simulink model "MagnetSystem"  (R2020b)
settings: Solver=VariableStepAuto  StartTime=0.0  StopTime=10  FixedStep=0.001  RelTol=1e-3
values from neighbouring files (symbols this model uses):
  A = [0, dfdx/m, dfdi/m ... (first row only)    [magnetABCD.m]
  B = [0 ... (first row only)    [magnetABCD.m]
  C = zeros(2,3)    [magnetABCD.m]
  x0 = positionConversion(equilibrium{ncards, 4})    [equilibriumFeatures.m]
undefined symbols (not defined in the file or in its folder): coeffLQR, coeffPP, current, F, initialConditions, initialConditionsOBS, intensityVariance, kdp, kic, kip, KoK, KoLQR, kpc, kpp, LL, positions, positionsVariance, target
libraries: simulink x1
settings Model: Creator=paolo  LastModifiedBy=paolo

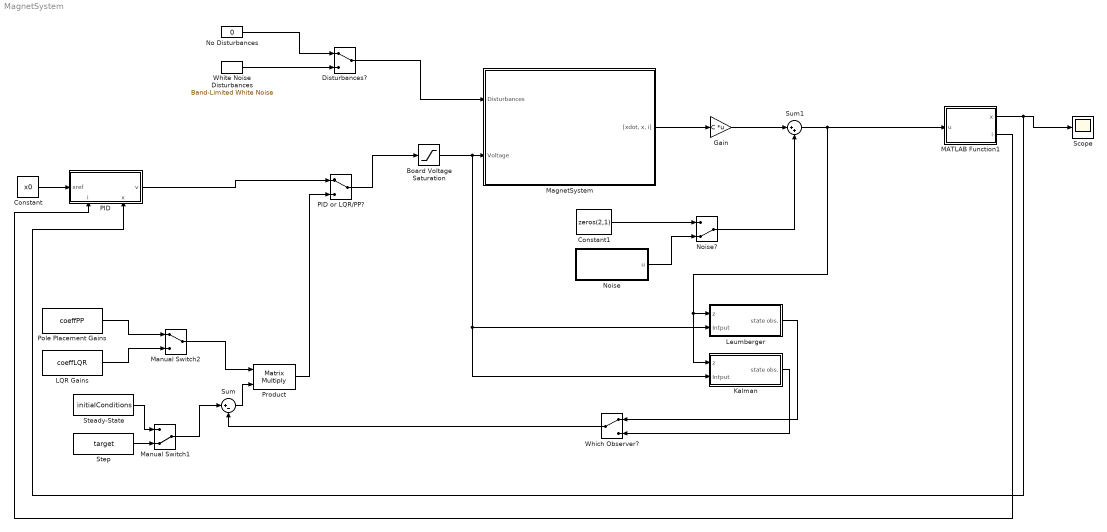
== system MagnetSystem ==
  Board Voltage Saturation : Saturate  UpperLimit=15  LowerLimit=0.1
  Constant : Constant  Value=x0
  Constant1 : Constant  Value=zeros(2,1)
  Disturbances? : ManualSwitch
  Gain : Gain  Gain=C  Multiplication=Matrix(K*u)
  Kalman : Subsystem
  LQR Gains : Constant  Value=coeffLQR  VectorParams1D=off
  Leumberger : Subsystem
  MATLAB Function1 : MATLAB Function  TreatAsAtomicUnit=on
  MagnetSystem : Subsystem
  Manual Switch1 : ManualSwitch  CurrentSetting=0
  Manual Switch2 : ManualSwitch
  No Disturbances : Constant  Value=0
  Noise : Subsystem
  Noise? : ManualSwitch  CurrentSetting=0
  PID : Subsystem
      settings: PortSchema="{\"entries\":[{\"content\":{\"sides\":[{\"content\":{\"connectorIds\":[\"In1\"]},\"type\":\"ConnectorPlacement.EquallySpacedRectSide\",\"uuid\":\"14521f87-e048-4244-bdcc-908d8d88763b\"},{\"content\":{\"connectorIds\":[\"Out1\"],\"side\":\"RIGHT\"},\"type\":\"ConnectorPlacement.EquallySpacedRectSide\",\"uuid\":\"c5527259-ae1a-43ba-91f2-6df4aeebe36b\"},{\"content\":{\"connectorIds\":[],\"side\":\"TOP\"},\"type\":\"ConnectorPlacement.EquallySpacedRectSide\",\"uuid\":\"73278f71-19a1-45c2-a1b8-f0fc113770d2\"},{\"content\":{\"connectorIds\":[\"In2\",\"In3\"],\"side\":\"BOTTOM\"},\"type\":\"ConnectorPlacement.EquallySpacedRectSide\",\"uuid\":\"a0ac4a62-b9ad-495a-a277-bc45d4b1109c\"},{\"content\":{\"connectorIds\":[],\"side\":\"HIDDEN\"},\"type\":\"ConnectorPlacement.EquallySpacedRectSide\",\"uuid\":\"850a1bc1-7bbe-470b-baa6-7596bfe1b42b\"}]},\"type\":\"ConnectorPlacement.EquallySpacedConnector\",\"uuid\":\"f2c623c1-bb11-4af5-93db-0114832c2495\"}],\"packageUris\":[\"http://schema.mathworks.com/mf0/Connector/R2020b\"],\"version\":\"1.0\"}"
  PID or LQR/PP? : ManualSwitch
  Pole Placement Gains : Constant  Value=coeffPP  VectorParams1D=off
  Product : Product  Multiplication=Matrix(*)
  Scope : Scope
  Steady-State : Constant  Value=initialConditions  VectorParams1D=off
  Step : Constant  Value=target  VectorParams1D=off
  Sum : Sum  Inputs=|+-
  Sum1 : Sum  Inputs=|++
  Which Observer? : ManualSwitch
  White Noise Disturbances : simulink/Sources/Band-Limited White Noise  Cov=[0.1]  Ts=0.1  seed=[23341]
  wires:
  Board Voltage Saturation/1 -> Kalman/2(Intput), Leumberger/2(Intput), MagnetSystem/2(Voltage)
  MagnetSystem/1("[xdot, x, i]") -> Gain/1
  Steady-State/1 -> Manual Switch1/1
  Sum/1 -> Product/2
  No Disturbances/1 -> Disturbances?/1
  Disturbances?/1 -> MagnetSystem/1(Disturbances)
  White Noise Disturbances/1 -> Disturbances?/2
  Step/1 -> Manual Switch1/2
  Manual Switch1/1 -> Sum/1
  Product/1 -> PID or LQR/PP?/2
  PID or LQR/PP?/1 -> Board Voltage Saturation/1
  PID/1(v) -> PID or LQR/PP?/1
  Constant/1 -> PID/1(xref)
  Manual Switch2/1 -> Product/1
  LQR Gains/1 -> Manual Switch2/2
  Pole Placement Gains/1 -> Manual Switch2/1
  Leumberger/1(state obs.) -> Which Observer?/1
  Kalman/1(state obs.) -> Which Observer?/2
  Which Observer?/1 -> Sum/2
  Gain/1 -> Sum1/1
  MATLAB Function1/1(x) -> PID/3(x), Scope/1
  Noise?/1 -> Sum1/2
  Noise/1(u) -> Noise?/2
  Sum1/1 -> Kalman/1(z), Leumberger/1(z), MATLAB Function1/1(u)
  Constant1/1 -> Noise?/1
  MATLAB Function1/2(i) -> PID/2(i)

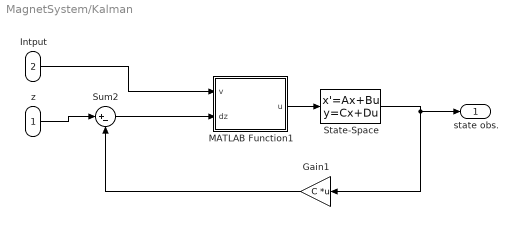
== system MagnetSystem/Kalman ==
  z : Inport
  Intput : Inport  Port=2
  Gain1 : Gain  Gain=C  Multiplication=Matrix(K*u)
  MATLAB Function1 : MATLAB Function  TreatAsAtomicUnit=on
  State-Space : StateSpace  A=A  B=[B KoK]  C=eye(3)  D=zeros(3,3)  InitialCondition=initialConditionsOBS
  Sum2 : Sum  Inputs=|+-
  state obs. : Outport
  wires:
  z/1 -> Sum2/1
  State-Space/1 -> Gain1/1, state obs./1
  Gain1/1 -> Sum2/2
  Sum2/1 -> MATLAB Function1/2(dz)
  Intput/1 -> MATLAB Function1/1(v)
  MATLAB Function1/1(u) -> State-Space/1

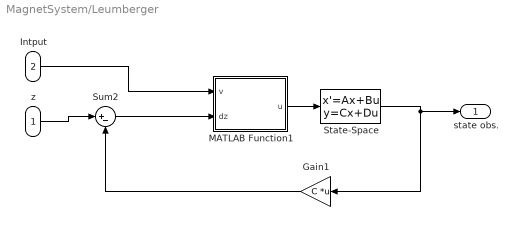
== system MagnetSystem/Leumberger ==
  z : Inport
  Intput : Inport  Port=2
  Gain1 : Gain  Gain=C  Multiplication=Matrix(K*u)
  MATLAB Function1 : MATLAB Function  TreatAsAtomicUnit=on
  State-Space : StateSpace  A=A  B=[B KoLQR]  C=eye(3)  D=zeros(3,3)  InitialCondition=initialConditionsOBS
  Sum2 : Sum  Inputs=|+-
  state obs. : Outport
  wires:
  z/1 -> Sum2/1
  State-Space/1 -> Gain1/1, state obs./1
  Gain1/1 -> Sum2/2
  Sum2/1 -> MATLAB Function1/2(dz)
  Intput/1 -> MATLAB Function1/1(v)
  MATLAB Function1/1(u) -> State-Space/1

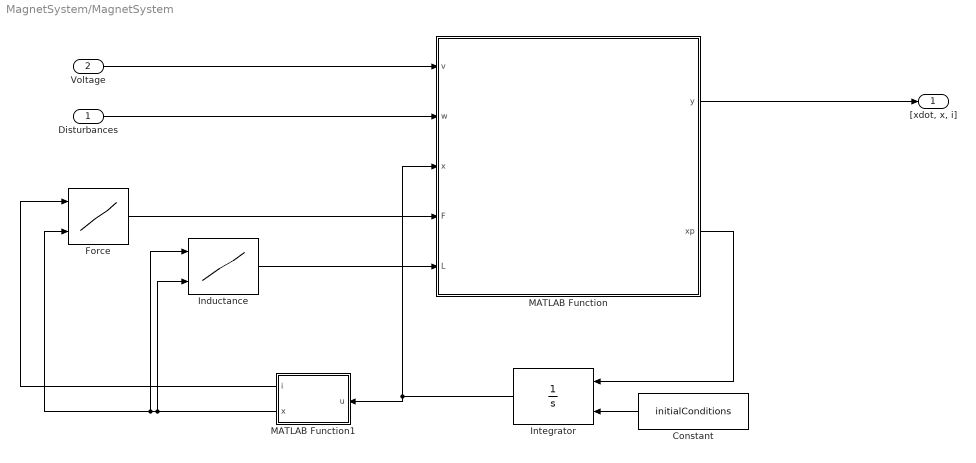
== system MagnetSystem/MagnetSystem ==
  Disturbances : Inport
  Voltage : Inport  Port=2
  Constant : Constant  Value=initialConditions
  Force : Lookup_n-D  BreakpointsForDimension1=current  BreakpointsForDimension2=positions  Table=F  InternalRulePriority=Speed  RndMeth=Simplest  InputSameDT=on
      settings: InputPortMap=u0,u1
  Inductance : Lookup_n-D  BreakpointsForDimension1=current  BreakpointsForDimension2=positions  Table=LL  InternalRulePriority=Speed  RndMeth=Simplest  InputSameDT=on
      settings: InputPortMap=u0,u1
  Integrator : Integrator  InitialConditionSource=external
  MATLAB Function : MATLAB Function  TreatAsAtomicUnit=on
  MATLAB Function1 : MATLAB Function  TreatAsAtomicUnit=on
  "[xdot, x, i]" : Outport
  wires:
  Integrator/1 -> MATLAB Function1/1(u), MATLAB Function/3(x)
  Voltage/1 -> MATLAB Function/1(v)
  Constant/1 -> Integrator/2
  Disturbances/1 -> MATLAB Function/2(w)
  MATLAB Function/1(y) -> "[xdot, x, i]"/1
  MATLAB Function/2(xp) -> Integrator/1
  MATLAB Function1/1(i) -> Force/1
  MATLAB Function1/2(x) -> Inductance/2, Force/2, Inductance/1
  Inductance/1 -> MATLAB Function/5(L)
  Force/1 -> MATLAB Function/4(F)

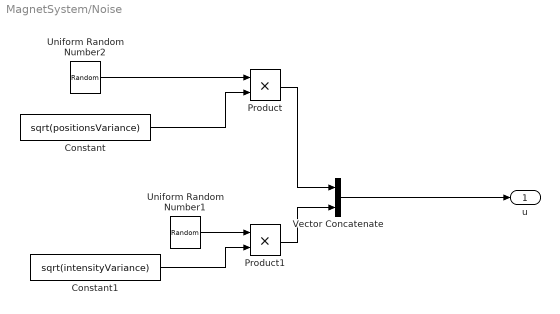
== system MagnetSystem/Noise ==
  Constant : Constant  Value=sqrt(positionsVariance)
  Constant1 : Constant  Value=sqrt(intensityVariance)
  Product : Product
  Product1 : Product
  Uniform Random Number1 : UniformRandomNumber  SampleTime=0.001
  Uniform Random Number2 : UniformRandomNumber  SampleTime=0.001
  Vector Concatenate : Concatenate  Mode=Multidimensional array
  u : Outport
  wires:
  Constant1/1 -> Product1/2
  Vector Concatenate/1 -> u/1
  Constant/1 -> Product/2
  Product1/1 -> Vector Concatenate/2
  Product/1 -> Vector Concatenate/1
  Uniform Random Number2/1 -> Product/1
  Uniform Random Number1/1 -> Product1/1

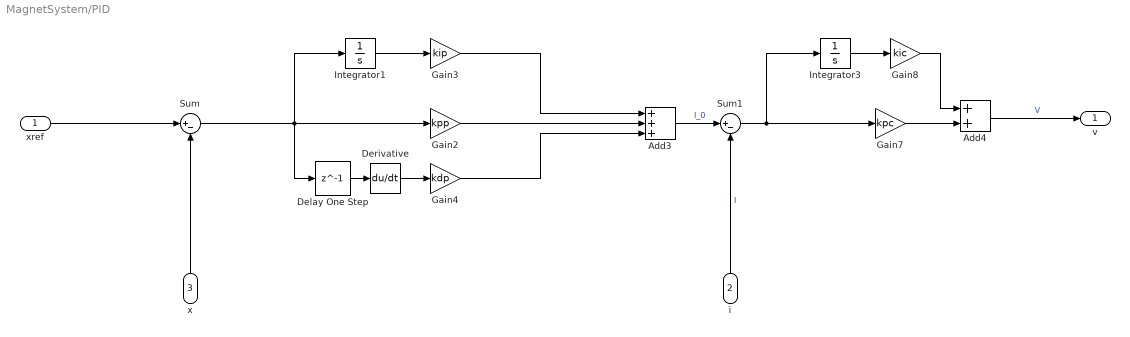
== system MagnetSystem/PID ==
  xref : Inport
  i : Inport  Port=2
  x : Inport  Port=3
  Add3 : Sum  Inputs=+++
  Add4 : Sum
  Delay One Step : Delay  DelayLength=1
  Derivative : Derivative
  Gain2 : Gain  Gain=kpp
  Gain3 : Gain  Gain=kip
  Gain4 : Gain  Gain=kdp
  Gain7 : Gain  Gain=kpc
  Gain8 : Gain  Gain=kic
  Integrator1 : Integrator
  Integrator3 : Integrator
  Sum : Sum  Inputs=|+-
  Sum1 : Sum  Inputs=|+-
  v : Outport
  wires:
  Sum/1 -> Integrator1/1, Delay One Step/1, Gain2/1
  Add4/1 -> v/1  "V"
  Gain4/1 -> Add3/3
  Derivative/1 -> Gain4/1
  i/1 -> Sum1/2  "I"
  Gain3/1 -> Add3/1
  Add3/1 -> Sum1/1  "I_0"
  Gain2/1 -> Add3/2
  Gain7/1 -> Add4/2
  Sum1/1 -> Integrator3/1, Gain7/1
  Gain8/1 -> Add4/1
  Integrator1/1 -> Gain3/1
  Integrator3/1 -> Gain8/1
  xref/1 -> Sum/1
  x/1 -> Sum/2
  Delay One Step/1 -> Derivative/1

== matlab function MagnetSystem/MATLAB Function1 ==
  data: i output; u input; x output
function [i, x] = fcn(u)
x = u(2);
i = u(3);

== matlab function MagnetSystem/MATLAB Function ==
  data: v input; y output; w input; x input; xp output; F input; L input
function [y,xp] = fcn(v,w,x,F,L)

R = 4.1;
m = 0.8766;
g = 9.81;

x1 = x(1);
x2 = x(2);
x3 = x(3);

xp = [((F/m)-g);x1;((v+w)-R*x3)/L];
y = [x1;x2;x3];

== matlab function MagnetSystem/MATLAB Function1 ==
  data: x output; i output; u input
function [x, i] = fcn(u)
x = u(1);
i = u(2);

== matlab function MagnetSystem/Leumberger/MATLAB Function1 ==
  data: u output; v input; dz input
function u  = fcn(v,dz)
ut = [v, dz(1), dz(2)];
u = ut';

== matlab function MagnetSystem/Kalman/MATLAB Function1 ==
  data: u output; v input; dz input
function u  = fcn(v,dz)
ut = [v, dz(1), dz(2)];
u = ut';
